simulink model "linear_sliding_mode"  (R2019b)
settings: Solver=VariableStepAuto  StartTime=0.0  StopTime=5  RelTol=1e-3
settings Model: Creator=Alien  LastModifiedBy=Alien
settings SolverCC: ZeroCrossAlgorithm=Adaptive
settings DebuggingCC: IgnoredZcDiagnostic=none

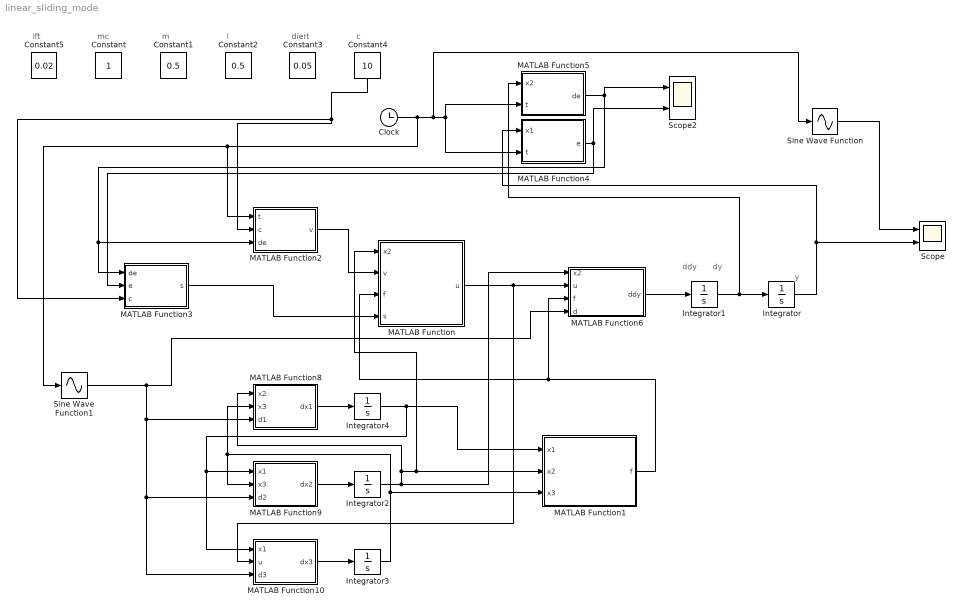
== system linear_sliding_mode ==
  note: c
  note: diert
  note: l
  note: m
  note: mc
  note: ddy
  note: dy
  note: y
  note: ift
  Clock : Clock
  Constant : Constant
  Constant1 : Constant  Value=0.5
  Constant2 : Constant  Value=0.5
  Constant3 : Constant  Value=0.05
  Constant4 : Constant  Value=10
  Constant5 : Constant  Value=0.02
  Integrator : Integrator  InitialCondition=0.15
  Integrator{1..4} (4 alike) : Integrator
  MATLAB Function : MATLAB Function  TreatAsAtomicUnit=on
  MATLAB Function1 : MATLAB Function  TreatAsAtomicUnit=on
  MATLAB Function10 : MATLAB Function  TreatAsAtomicUnit=on
  MATLAB Function2 : MATLAB Function  TreatAsAtomicUnit=on
  MATLAB Function3 : MATLAB Function  TreatAsAtomicUnit=on
  MATLAB Function4 : MATLAB Function  TreatAsAtomicUnit=on
  MATLAB Function5 : MATLAB Function  TreatAsAtomicUnit=on
  MATLAB Function6 : MATLAB Function  TreatAsAtomicUnit=on
  MATLAB Function8 : MATLAB Function  TreatAsAtomicUnit=on
  MATLAB Function9 : MATLAB Function  TreatAsAtomicUnit=on
  Scope : Scope  NumInputPorts=2
  Scope2 : Scope  NumInputPorts=2
  Sine Wave Function : Sin  TimeSource=Use external signal  SampleTime=0
  Sine Wave Function1 : Sin  TimeSource=Use external signal  Frequency=2*pi  SampleTime=0
  wires:
  Integrator1/1 -> MATLAB Function5/1(x2), Integrator/1
  MATLAB Function6/1(ddy) -> Integrator1/1
  MATLAB Function5/1(de) -> MATLAB Function2/3(de), MATLAB Function3/1(de), Scope2/1
  MATLAB Function4/1(e) -> MATLAB Function3/2(e), Scope2/2
  Constant4/1 -> MATLAB Function2/2(c), MATLAB Function3/3(c)
  Clock/1 -> Sine Wave Function1/1, MATLAB Function2/1(t), Sine Wave Function/1, MATLAB Function4/2(t), MATLAB Function5/2(t)
  MATLAB Function10/1(dx3) -> Integrator3/1
  MATLAB Function9/1(dx2) -> Integrator2/1
  Integrator2/1 -> MATLAB Function6/1(x2), MATLAB Function/1(x2), MATLAB Function1/2(x2), MATLAB Function8/1(x2)
  Integrator3/1 -> MATLAB Function1/3(x3), MATLAB Function9/2(x3), MATLAB Function8/2(x3)
  MATLAB Function/1(u) -> MATLAB Function10/2(u), MATLAB Function6/2(u)
  MATLAB Function8/1(dx1) -> Integrator4/1
  Integrator4/1 -> MATLAB Function10/1(x1), MATLAB Function9/1(x1), MATLAB Function1/1(x1)
  MATLAB Function1/1(f) -> MATLAB Function6/3(f), MATLAB Function/3(f)
  Integrator/1 -> Scope/2, MATLAB Function4/1(x1)
  MATLAB Function2/1(v) -> MATLAB Function/2(v)
  MATLAB Function3/1(s) -> MATLAB Function/4(s)
  Sine Wave Function/1 -> Scope/1
  Sine Wave Function1/1 -> MATLAB Function10/3(d3), MATLAB Function9/3(d2), MATLAB Function8/3(d1), MATLAB Function6/4(d)

== matlab function linear_sliding_mode/MATLAB Function1 ==
  data: x1 input; f output; x2 input; x3 input
function f = fcn(x1, x2, x3)
f = (x1^5 + x3)*(x3 + cos(x2)) + (x2 + 1)*x1^2;

== matlab function linear_sliding_mode/MATLAB Function ==
  data: x2 input; v input; u output; f input; s input
function u = fcn(x2, v, f, s)
nta = 3;
u = 1/(x2 + 1)*(v - f + nta*sign(s));

== matlab function linear_sliding_mode/MATLAB Function2 ==
  data: t input; v output; c input; de input
function v = fcn(t, c ,de)
v = -sin(t) + c*de;

== matlab function linear_sliding_mode/MATLAB Function3 ==
  data: de input; s output; e input; c input
function s = fcn(de, e, c)
s = de + c*e;

== matlab function linear_sliding_mode/MATLAB Function4 ==
  data: x1 input; e output; t input
function e = fcn(x1, t)
e = sin(t) - x1;

== matlab function linear_sliding_mode/MATLAB Function5 ==
  data: x2 input; de output; t input
function de = fcn(x2, t)
de = cos(t) - x2;

== matlab function linear_sliding_mode/MATLAB Function6 ==
  data: x2 input; u input; f input; ddy output; d input
function ddy = fcn(x2, u, f, d)
ddy = (x2 +1)*u + f + d;

== matlab function linear_sliding_mode/MATLAB Function8 ==
  data: x2 input; dx1 output; x3 input; d1 input
function dx1 = fcn(x2, x3, d1)
dx1 = sin(x2) + (x2 + 1)*x3 +d1;

== matlab function linear_sliding_mode/MATLAB Function9 ==
  data: x1 input; dx2 output; x3 input; d2 input
function dx2 = fcn(x1, x3, d2)
dx2 = x1^5+ x3 + d2;

== matlab function linear_sliding_mode/MATLAB Function10 ==
  data: x1 input; u input; dx3 output; d3 input
function dx3 = fcn(x1, u, d3)
dx3 = x1^2 + u + d3;
